simulink model "iterative_motion_controller_2023a"  (R2023a)
settings: Solver=FixedStepDiscrete  StartTime=0.0  StopTime=10.0  RelTol=1e-3
settings Model: DataDictionary=amcfoc.sldd  Creator=mfussi  LastModifiedBy=mfussi
settings SolverCC: AutoInsertRateTranBlk=on  InsertRTBMode=Never (minimum delay)
settings DataIOCC: SaveOutput=off  SignalLogging=off  DSMLogging=off  SaveTime=off  ReturnWorkspaceOutputs=off
settings OptimizationCC: DefaultParameterBehavior=Inlined  UseDivisionForNetSlopeComputation=on  UseFloatMulNetSlope=on  DefaultUnderspecifiedDataType=single  EnhancedBackFolding=on  PassReuseOutputArgsAs=Individual arguments  ZeroExternalMemoryAtStartup=off  ZeroInternalMemoryAtStartup=off  OptimizeBlockOrder=speed  DifferentSizesBufferReuse=on  OptimizationCustomize=off  EfficientTunableParamExpr=on
settings DebuggingCC: ParameterTunabilityLossMsg=error
settings HardwareCC: ProdBitPerPointer=32  ProdBitPerSizeT=32  ProdBitPerPtrDiffT=32  ProdLargestAtomicInteger=Long  ProdLargestAtomicFloat=Double  ProdWordSize=32  ProdLongLongMode=on  ProdHWDeviceType=ARM Compatible->ARM Cortex-M
settings SFSimCC: MATLABDynamicMemAlloc=off
settings RTWCC: Description=Embedded Coder  SystemTargetFile=ert.tlc  GenCodeOnly=on  TemplateMakefile=ert_default_tmf
settings CodeAppCC: ForceParamTrailComments=on  IgnoreCustomStorageClasses=off  MaxIdLength=60  OperatorAnnotations=on  SimulinkDataObjDesc=on  SFDataObjDesc=on  InsertBlockDesc=on
settings ERTTargetCC: TargetLangStandard=C99 (ISO)  CodeReplacementLibrary=ARM Cortex-M,iCubTech  GenerateSampleERTMain=on  InlinedParameterPlacement=NonHierarchical  ERTCustomFileTemplate=example_file_process.tlc

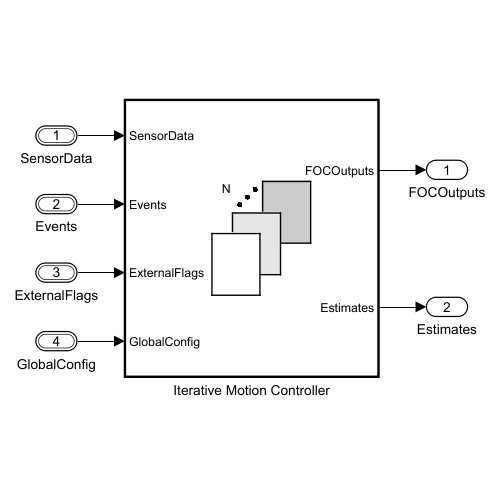
[thumbnail: Simulink's stored preview of the top-level diagram]
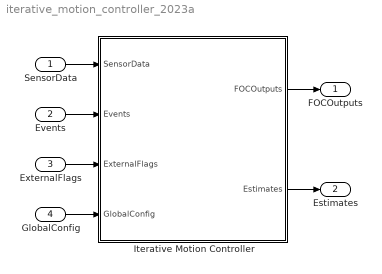
== system iterative_motion_controller_2023a ==
  SensorData : Inport  OutDataTypeStr=Bus: SensorsData  PortDimensions=numberOfActuators  BusOutputAsStruct=on
  Events : Inport  Port=2  OutDataTypeStr=Bus: SupervisorReceivedEvents  PortDimensions=numberOfActuators  BusOutputAsStruct=on
  ExternalFlags : Inport  Port=3  OutDataTypeStr=Bus: ExternalFlags  BusOutputAsStruct=on
  GlobalConfig : Inport  Port=4  OutDataTypeStr=Bus: GlobalConfiguration  BusOutputAsStruct=on
  Iterative Motion Controller : Subsystem  TreatAsAtomicUnit=on
  FOCOutputs : Outport  PortDimensions=numberOfActuators
  Estimates : Outport  Port=2  PortDimensions=numberOfActuators
  wires:
  SensorData/1 -> Iterative Motion Controller/1(SensorData)
  Iterative Motion Controller/1(FOCOutputs) -> FOCOutputs/1
  Iterative Motion Controller/2(Estimates) -> Estimates/1
  Events/1 -> Iterative Motion Controller/2(Events)
  ExternalFlags/1 -> Iterative Motion Controller/3(ExternalFlags)
  GlobalConfig/1 -> Iterative Motion Controller/4(GlobalConfig)

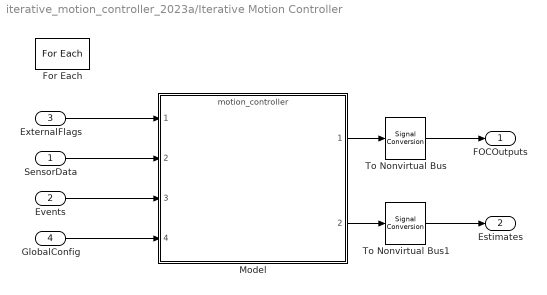
== system iterative_motion_controller_2023a/Iterative Motion Controller ==
  SensorData : Inport  Partition=on  PartitionDimension=1  PartitionWidth=1  PartitionOffset=0
  Events : Inport  Port=2  Partition=on  PartitionDimension=1  PartitionWidth=1  PartitionOffset=0
  ExternalFlags : Inport  Port=3
  GlobalConfig : Inport  Port=4
  For Each : ForEach  DisableCoverage=on
  Model : ModelReference  ModelNameDialog=motion_controller.slx  ModelReferenceVersion=2.156
  To Nonvirtual Bus : SignalConversion  ConversionOutput=Nonvirtual bus  OverrideOpt=off
  To Nonvirtual Bus1 : SignalConversion  ConversionOutput=Nonvirtual bus  OverrideOpt=off
  FOCOutputs : Outport  OutDataTypeStr=Bus: FOCOutputs  ConcatenationDimension=1
  Estimates : Outport  Port=2  OutDataTypeStr=Bus: EstimatedData  ConcatenationDimension=1
  wires:
  SensorData/1 -> Model/2
  Events/1 -> Model/3
  Model/1 -> To Nonvirtual Bus/1
  Model/2 -> To Nonvirtual Bus1/1
  ExternalFlags/1 -> Model/1
  GlobalConfig/1 -> Model/4
  To Nonvirtual Bus/1 -> FOCOutputs/1
  To Nonvirtual Bus1/1 -> Estimates/1
